simulink model "EV_thermal_charger_2015a_jmaab_Can01"  (R2015a)
settings: Solver=ode3  StartTime=0.0  StopTime=1800  FixedStep=sampling_time  RelTol=1e-3
PreLoadFcn:
  | %run('init_setting.m')
PostLoadFcn:
  | %set_param(gcs, 'SimulationCommand', 'update');
  | %load('save_param/save_P_Charger', 'P_Charger');
  | %load('save_param/save_T_User_set_temp_degC','T_User_set_temp_degC');
  | %load('save_param/save_ENV_PNT_PTTH_Temp_add_degC','ENV_PNT_PTTH_Temp_add_degC');
  | %load('save_param/save_ENV_PNT_CABIN_Temp_add_degC','ENV_PNT_CABIN_Temp_add_degC');
  | %load('save_param/save_ENV_PNT_PHI_Sunlight_W','ENV_PNT_PHI_Sunlight_W');
  | %load('save_param/save_ENV_PNT_Outside_Temp_ini_degC','ENV_PNT_Outside_Temp_ini_degC');
undefined symbols (not defined in the file or in its folder): BK_PNT_Pow_UL, BK_PNT_ReGene_vel_limit_DN_kmph, BK_PNT_ReGene_vel_limit_UP_kmph, BK_PNT_Tau_brake, Brk_LL, Brk_PGain, Brk_UL, BT_PNT_Hi_C_pol_hi_batt, BT_PNT_Hi_Capa_hi_batt_F, BT_PNT_Hi_ocv_SOC_hi_batt_OCV_V_table, BT_PNT_Hi_ocv_SOC_hi_batt_OCV_V_table_x_SOC, BT_PNT_Hi_R_hi_batt_cell, BT_PNT_Hi_R_pol_hi_batt, BT_PNT_Hi_SOC_MAX_hi_batt, BT_PNT_Hi_SOC_MIN_hi_batt, BT_PNT_Hi_SOC_START_hi_batt, BT_PNT_Lo_Capa_lo_batt_F, BT_PNT_Lo_ocv_SOC_lo_batt_OCV_V_table, BT_PNT_Lo_ocv_SOC_lo_batt_OCV_V_table_x_SOC, BT_PNT_Lo_R_lo_batt_ohm, BT_PNT_Lo_SOC_MAX_lo_batt, BT_PNT_Lo_SOC_MIN_lo_batt, BT_PNT_Lo_SOC_START_lo_batt, BTTH_CNT_P_BT_Heater_W, BTTH_CNT_P_BT_Heater_W_x_BTCells_degC, BTTH_CNT_Voltage_BTFan_V, BTTH_CNT_Voltage_BTFan_V_x_BTCells_degC, BTTH_PNT_BT_Heat_Resi_KpW, BTTH_PNT_BT_Heat_Resi_KpW_x_Wind_m3ps, BTTH_PNT_BT_Heater2BTCells_Heat_Resi_KpW, BTTH_PNT_BT_Heater_Heat_Capa_JpK, BTTH_PNT_BTBlock2BTAir_Heat_Resi_KpW, BTTH_PNT_BTBlock_Heat_Capa_JpK, BTTH_PNT_BTCells2BTBlock_Heat_Resi_KpW, BTTH_PNT_BTCells_Heat_Capa_JpK, BTTH_PNT_v_BTFan_Wind_vel_mps, BTTH_PNT_v_BTFan_Wind_vel_mps_x_V_BTFan, CATH_CNT_P_Aircon_W_LL, CATH_CNT_P_Aircon_W_UL, CATH_CNT_P_Gain_Aircon, CATH_CNT_P_Gain_PTC_Heater, CATH_CNT_P_Gain_SeatHT, CATH_CNT_P_PTC_Heater, CATH_CNT_P_PTC_Heater_W_LL, CATH_CNT_P_PTC_Heater_W_UL, CATH_CNT_P_PTC_Heater_x_T_Outside_temp_degC, CATH_CNT_P_SeatHT_W_LL, CATH_CNT_P_SeatHT_W_UL, CATH_CNT_PGain_Temp_blowout, CATH_CNT_T_Aircon_Indoor_degC, CATH_CNT_T_Aircon_Indoor_degC_x_T_blowout_degC, CATH_CNT_T_PTC_Heater_degC_UL, CATH_CNT_T_SeatHT_Temp_degC, CATH_CNT_T_SeatHT_Temp_degC_x_T_blowout_degC, CATH_CNT_V_HVAC_Fan, CATH_CNT_V_HVAC_Fan_x_T_blowout_degC, CATH_CNT_V_RDFan_V, CATH_CNT_V_RDFan_x_P_Aircon_W, CATH_PNT_Air_Convection_Heat_Resi_KpW, CATH_PNT_Air_Convection_Heat_Resi_x_mps ... (+141)
undefined symbols (not defined in the file): ACC_D_Gain, ACC_I_Gain, ACC_P_Gain
libraries: METI_Lib_vehicle_model x52, simulink x35
(part 5 of 6)

== system EV_thermal_charger_2015a_jmaab_Can01/Vehicle/CNT/VCU_CNT/VCU_CNT/PDfSOC ==
  note: 放電電力マップ
  note: 充電電力マップ
  SOC_BT_Hi_PNT_per : Inport
  PSoFin_map : Lookup_n-D  NumberOfTableDimensions=1  BreakpointsForDimension1=VCU_CNT_PSoFin_soc  BeginIndexSearchUsingPreviousIndexResult=on  Table=VCU_CNT_PSoFin_battpw  ExtrapMethod=Clip  UseLastTableValue=on  InternalRulePriority=Speed  RndMeth=Simplest  InputSameDT=on
  PSoFout_map : Lookup_n-D  NumberOfTableDimensions=1  BreakpointsForDimension1=VCU_CNT_PSoFout_soc  BeginIndexSearchUsingPreviousIndexResult=on  Table=VCU_CNT_PSoFout_battpw  ExtrapMethod=Clip  UseLastTableValue=on  InternalRulePriority=Speed  RndMeth=Simplest  InputSameDT=on
  PSoFin : Outport
  PSoFout : Outport  Port=2
  wires:
  PSoFout_map/1 -> PSoFout/1
  PSoFin_map/1 -> PSoFin/1
  SOC_BT_Hi_PNT_per/1 -> PSoFout_map/1, PSoFin_map/1

== system EV_thermal_charger_2015a_jmaab_Can01/Vehicle/CNT/VCU_CNT/VCU_CNT/ReGenerativeBrake_Calc ==
  note: 回生ブレーキ
      | 推進力[N]
  note: 回生ブレーキ
      | モータートルク[N]
  v_VL_PNT_kmph : Inport
  open_break_Driver_per : Inport  Port=2
  Constant : Constant  Value=0
  Constant2 : Constant  Value=1/TM_PNT_ratio_MG2_gear
  Constant4 : Constant  Value=tire_r
  Constant5 : Constant  Value=BK_PNT_Pow_UL
  Constant9 : Constant  Value=1/DF_PNT_DF_gear
  Gain : Gain  Gain=-1
  Product1 : Product  Inputs=6
  Product2 : Product
  ReBrake_Limit_Lowspeed : Subsystem
  Saturation Dynamic : simulink/Discontinuities/Saturation Dynamic  OutMin=[]  OutMax=[]  OutDataTypeStr=Inherit: Same as second input  OutDataType=fixdt(1, 16)  OutScaling=2^-10  DoSatur=off
  eta_DF1 : Constant  Value=TM_PNT_eta_MG2_gear
  eta_DF2 : Constant  Value=DF_PNT_eta_DF
  per2F2 : Gain  Gain=1/100
  trq_R_brake_tgt : Outport
  wires:
  Saturation Dynamic/1 -> Product1/1
  Constant/1 -> Saturation Dynamic/1
  Gain/1 -> Saturation Dynamic/2
  per2F2/1 -> Product2/1
  Constant5/1 -> Product2/2
  Product2/1 -> Gain/1
  open_break_Driver_per/1 -> per2F2/1
  Constant4/1 -> Product1/2
  Constant9/1 -> Product1/3
  eta_DF2/1 -> Product1/4
  Product1/1 -> trq_R_brake_tgt/1
  Constant2/1 -> Product1/5
  eta_DF1/1 -> Product1/6
  v_VL_PNT_kmph/1 -> ReBrake_Limit_Lowspeed/1(v_VL_PNT_kmph)
  ReBrake_Limit_Lowspeed/1(F_Brake_limit_lowspeed) -> Saturation Dynamic/3

== system EV_thermal_charger_2015a_jmaab_Can01/Vehicle/CNT/VCU_CNT/VCU_CNT/trq_MG2_GuardCalc ==
  note: 回生側のトルク制限
  note: 加速側のトルク制限
  w_MG_PNT_radps : Inport
  PSoFin : Inport  Port=2
  PSoFout : Inport  Port=3
  P_HVAC_PNT_W : Inport  Port=4
  P_DCDC_PNT_W : Inport  Port=5
  Abs : Abs
  Divide_0wari : METI_Lib_vehicle_model/Divide_0wari
  Divide_0wari1 : METI_Lib_vehicle_model/Divide_0wari
  MinMax : MinMax  Function=max  Inputs=2
  MinMax1 : MinMax  Inputs=2
  MinMax2 : MinMax  Inputs=2
  MinMax3 : MinMax  Function=max  Inputs=2
  Subtract1 : Sum  Inputs=+--
  Subtract2 : Sum  Inputs=+--
  力行側出力上限 : Constant  Value=MG_CNT_Pmax_MG_Gene_W
  力行側定トルク回転数上限 : Constant  Value=MG_CNT_MG_Const_trq_Gene_radps
  回生側出力上限 : Constant  Value=MG_CNT_Pmin_MG_ReGene_W
  回生側定トルク回転数上限 : Constant  Value=MG_CNT_MG_Const_trq_ReGene_radps
  trq_MG2_UpperGuard : Outport
  trq_MG2_LowerGuard : Outport  Port=2
  wires:
  MinMax2/1 -> Divide_0wari1/1  "使用可能電力"
  w_MG_PNT_radps/1 -> Abs/1
  Divide_0wari1/1 -> trq_MG2_UpperGuard/1  "トルク上限"
  MinMax/1 -> Divide_0wari1/2, Divide_0wari/2
  Abs/1 -> MinMax/1
  MinMax1/1 -> MinMax/2
  PSoFout/1 -> Subtract1/1  "バッテリ放電電力上限値"
  P_HVAC_PNT_W/1 -> Subtract2/2, Subtract1/2
  MinMax3/1 -> Divide_0wari/1
  Divide_0wari/1 -> trq_MG2_LowerGuard/1
  PSoFin/1 -> Subtract2/1
  力行側定トルク回転数上限/1 -> MinMax1/1
  回生側定トルク回転数上限/1 -> MinMax1/2
  Subtract1/1 -> MinMax2/1  "使用可能電力"
  Subtract2/1 -> MinMax3/2
  力行側出力上限/1 -> MinMax2/2
  回生側出力上限/1 -> MinMax3/1
  P_DCDC_PNT_W/1 -> Subtract2/3, Subtract1/3

== system EV_thermal_charger_2015a_jmaab_Can01/Vehicle/CNT/VCU_CNT/VCU_CNT/trq_MG2_tgtCalc2 ==
  note: ～回生協調ブレーキ時～
      | アクセルオフによる回生ブレーキトルクと
      | ブレーキ操作による回生ブレーキトルクを合算し
      | モーター要求トルクとする
  note: ～回生協調ブレーキ時～
      | モーター要求トルクから
      | アクセルオフによる回生ブレーキトルクを減算し
      | 実際に出力できているブレーキ操作による回生ブレーキトルクを算出
      | それを車両駆動力としてブレーキECUへ送信する
  User_Power_req : Inport
  w_MG_PNT_radps : Inport  Port=2
  trq_motor_UserAcc_tgt : Inport  Port=3
  trq_MG2_UpperGuard : Inport  Port=4
  trq_MG2_LowerGuard : Inport  Port=5
  trq_R_brake_tgt : Inport  Port=6
  Add : Sum
  Add1 : Sum  Inputs=+-
  Constant1 : Constant  Value=TM_PNT_ratio_MG2_gear
  Constant2 : Constant  Value=DF_PNT_DF_gear
  Constant4 : Constant  Value=1/tire_r
  Product1 : Product  Inputs=6
  Saturation Dynamic2 : simulink/Discontinuities/Saturation Dynamic  OutMin=[]  OutMax=[]  OutDataTypeStr=Inherit: Same as second input  OutDataType=fixdt(1, 16)  OutScaling=2^-10  DoSatur=off
  Saturation Dynamic4 : simulink/Discontinuities/Saturation Dynamic  OutMin=[]  OutMax=[]  OutDataTypeStr=Inherit: Same as second input  OutDataType=fixdt(1, 16)  OutScaling=2^-10  DoSatur=off
  Switch4 : Switch  Criteria=u2 > Threshold
  eta_DF1 : Constant  Value=1/DF_PNT_eta_DF
  eta_DF2 : Constant  Value=1/TM_PNT_eta_MG2_gear
  回転数上限超過時トルク制限処理 : Subsystem
  tgt_Trq_VCU_CNT_MG_Nm : Outport
  F_VCU_CNT_re_break_N : Outport  Port=2
  wires:
  Saturation Dynamic4/1 -> Add1/1, tgt_Trq_VCU_CNT_MG_Nm/1
  trq_MG2_LowerGuard/1 -> Saturation Dynamic2/3, Saturation Dynamic4/3
  回転数上限超過時トルク制限処理/1(flag_overrev) -> Switch4/2
  Add/1 -> Saturation Dynamic4/2
  trq_motor_UserAcc_tgt/1 -> 回転数上限超過時トルク制限処理/1(trq_MG2_tgt), Switch4/1
  trq_MG2_UpperGuard/1 -> Saturation Dynamic2/1, Saturation Dynamic4/1
  w_MG_PNT_radps/1 -> 回転数上限超過時トルク制限処理/2(w_ROT_motor)
  User_Power_req/1 -> 回転数上限超過時トルク制限処理/3(User_Power_req)
  回転数上限超過時トルク制限処理/2(trq_MG2_guarded) -> Switch4/3
  Add1/1 -> Product1/1
  Constant4/1 -> Product1/2
  Constant2/1 -> Product1/3
  eta_DF1/1 -> Product1/4
  Product1/1 -> F_VCU_CNT_re_break_N/1
  Switch4/1 -> Add/2, Saturation Dynamic2/2
  trq_R_brake_tgt/1 -> Add/1
  Saturation Dynamic2/1 -> Add1/2
  Constant1/1 -> Product1/5
  eta_DF2/1 -> Product1/6

== system EV_thermal_charger_2015a_jmaab_Can01/Vehicle/CNT/VCU_CNT/VCU_CNT/ユーザ要求駆力算出 ==
  note: 低速時に目標出力が0にならないよう
      | 5km/h以下では車速を5km/hとして
      | 目標出力を計算するための
      | 速度切替処理
  note: モーター軸の要求トルク
  open_accel_Driver_per : Inport
  open_break_Driver_per : Inport  Port=2
  v_VL_PNT_kmph : Inport  Port=3
  Compare To Constant : simulink/Logic and Bit Operations/Compare To Constant  relop=<  const=VCU_CNT_trq_req_v_vehicle_th  OutDataTypeStr=boolean
  Compare To Constant1 : simulink/Logic and Bit Operations/Compare To Constant  relop=>  const=VCU_CNT_trq_req_brak_th  OutDataTypeStr=boolean
  Constant : Constant  Value=5
  Constant1 : Constant  Value=DF_PNT_DF_gear
  Constant2 : Constant  Value=TM_PNT_ratio_MG2_gear
  Constant3 : Constant  Value=VCU_CNT_trq_req_Gain_ON
  Constant4 : Constant  Value=1/tire_r
  Constant5 : Constant  Value=VCU_CNT_trq_req_Gain_OFF
  Gain1 : Gain  Commented=through  Gain=mps2kmph
  Logical Operator : Logic  AllPortsSameDT=off  OutDataTypeStr=boolean
  Product : Product
  Product1 : Product  Inputs=6
  Product3 : Product
  Relational Operator : RelationalOperator  Operator=>  OutDataTypeStr=boolean
  Switch : Switch  Criteria=u2 > Threshold  Threshold=0.5
  Switch1 : Switch  Criteria=u2 > Threshold  Threshold=0.5
  Transfer Fcn : TransferFcn  Denominator=[VCU_CNT_trq_req_delaytime 1]
  eta_DF1 : Constant  Value=DF_PNT_eta_DF
  eta_DF2 : Constant  Value=TM_PNT_eta_MG2_gear
  kmph2mps : Gain  Gain=kmph2mps
  kmph2mps1 : Gain  Commented=through  Gain=kmph2mps
  mps2kmph : Gain  Commented=through  Gain=mps2kmph
  要求駆動トルク推定 : Lookup_n-D  BreakpointsForDimension1=VCU_CNT_trq_require_v_kmph  BreakpointsForDimension2=VCU_CNT_trq_require_accper  BeginIndexSearchUsingPreviousIndexResult=on  Table=VCU_CNT_trq_require_Nm  ExtrapMethod=Clip  InternalRulePriority=Speed  RndMeth=Simplest  InputSameDT=on
  P_vehicle_tgt : Outport
  trq_motor_UserAcc_tgt : Outport  Port=2
  wires:
  Switch/1 -> kmph2mps/1
  Product3/1 -> P_vehicle_tgt/1
  Constant/1 -> kmph2mps1/1, Relational Operator/2
  mps2kmph/1 -> Relational Operator/1
  Relational Operator/1 -> Switch/2
  kmph2mps1/1 -> Switch/3
  Constant4/1 -> Product1/1
  Constant1/1 -> Product1/2
  eta_DF1/1 -> Product1/3
  Product1/1 -> Product3/2
  要求駆動トルク推定/1 -> Product1/6, Product/1
  Constant5/1 -> Switch1/1
  v_VL_PNT_kmph/1 -> mps2kmph/1, Gain1/1, Switch/1
  open_break_Driver_per/1 -> Compare To Constant1/1
  Compare To Constant/1 -> Logical Operator/1
  Compare To Constant1/1 -> Logical Operator/2
  Logical Operator/1 -> Switch1/2
  Constant3/1 -> Switch1/3
  Switch1/1 -> Transfer Fcn/1
  Transfer Fcn/1 -> Product/2
  Product/1 -> trq_motor_UserAcc_tgt/1
  Gain1/1 -> 要求駆動トルク推定/1, Compare To Constant/1
  open_accel_Driver_per/1 -> 要求駆動トルク推定/2
  Constant2/1 -> Product1/4
  eta_DF2/1 -> Product1/5
  kmph2mps/1 -> Product3/1

== system EV_thermal_charger_2015a_jmaab_Can01/Vehicle/DTTH/DTTH_PNT/DFTH_PNT/DFBlock2Air_Heat_Resistance ==
  "T_DFBlock_Resi3_K " : Inport
  T_DF_Air_Resi1_K : Inport  Port=2
  Add : Sum  Inputs=+-
  Constant : Constant  Value=PTTH_PNT_DFBlock2DFAir_Heat_Resi_KpW
  Divide : Product  Inputs=*/
  Gain : Gain  Gain=-1
  Gain1 : Gain
  "PHI_DF_Air_Resi1_W " : Outport
  "PHI_DFBlock_Resi3_W " : Outport  Port=2
  wires:
  Constant/1 -> Divide/2
  Add/1 -> Divide/1
  Divide/1 -> Gain/1, Gain1/1
  "T_DFBlock_Resi3_K "/1 -> Add/1
  Gain1/1 -> "PHI_DF_Air_Resi1_W "/1
  T_DF_Air_Resi1_K/1 -> Add/2
  Gain/1 -> "PHI_DFBlock_Resi3_W "/1

== system EV_thermal_charger_2015a_jmaab_Can01/Vehicle/DTTH/DTTH_PNT/DFTH_PNT/DFBlock_Heat_Capacity ==
  Temp_ini : Inport
  "PHI_DFBlock1_W " : Inport  Port=2
  "PHI_DFBlock2_W " : Inport  Port=3
  PHI_DFBlock3_W : Inport  Port=4
  Add : Sum  Inputs=+++
  Add1 : Sum
  Constant : Constant  Value=PTTH_PNT_DFBlock_Heat_Capa_JpK
  Divide : Product  Inputs=/*
  Integrator : Integrator
  degC->K : Subsystem
  "T_DFBlock1_K " : Outport
  T_DFBlock2_K : Outport  Port=2
  "T_DFBlock3_K " : Outport  Port=3
  wires:
  "PHI_DFBlock1_W "/1 -> Add/1
  Constant/1 -> Divide/1
  Add/1 -> Divide/2
  Divide/1 -> Integrator/1
  Temp_ini/1 -> degC->K/1(degC)
  Integrator/1 -> Add1/2
  Add1/1 -> "T_DFBlock3_K "/1, "T_DFBlock1_K "/1, T_DFBlock2_K/1
  "PHI_DFBlock2_W "/1 -> Add/2
  PHI_DFBlock3_W/1 -> Add/3
  degC->K/1(K) -> Add1/1

== system EV_thermal_charger_2015a_jmaab_Can01/Vehicle/DTTH/DTTH_PNT/DFTH_PNT/DFOil2DFBlock_Heat_Resistance ==
  T_DFBlock_Resi1_K : Inport
  "T_DFOil_Resi2_K " : Inport  Port=2
  Add : Sum  Inputs=+-
  Constant : Constant  Value=PTTH_PNT_DFOil2DFBlock_Heat_Resi_KpW
  Divide : Product  Inputs=*/
  Gain : Gain  Gain=-1
  Gain1 : Gain
  PHI_DFBlock_Resi1_W : Outport
  PHI_DFOil_Resi2_W : Outport  Port=2
  wires:
  Constant/1 -> Divide/2
  Add/1 -> Divide/1
  Divide/1 -> Gain1/1, Gain/1
  Gain/1 -> PHI_DFOil_Resi2_W/1
  "T_DFOil_Resi2_K "/1 -> Add/1
  T_DFBlock_Resi1_K/1 -> Add/2
  Gain1/1 -> PHI_DFBlock_Resi1_W/1

== system EV_thermal_charger_2015a_jmaab_Can01/Vehicle/DTTH/DTTH_PNT/DFTH_PNT/DFOil_Heat_Capacity ==
  Temp_ini : Inport
  PHI_DFOil1_W : Inport  Port=2
  "PHI_DFOil2_W " : Inport  Port=3
  Add : Sum
  Add1 : Sum
  Constant : Constant  Value=PTTH_PNT_DFOil_Heat_Capa_JpK
  Divide : Product  Inputs=/*
  Integrator : Integrator
  degC->K : Subsystem
  "T_DFOil1_K " : Outport
  T_DFOil2_K : Outport  Port=2
  wires:
  "PHI_DFOil2_W "/1 -> Add/2
  PHI_DFOil1_W/1 -> Add/1
  Constant/1 -> Divide/1
  Add/1 -> Divide/2
  Divide/1 -> Integrator/1
  Temp_ini/1 -> degC->K/1(degC)
  Integrator/1 -> Add1/2
  Add1/1 -> T_DFOil2_K/1, "T_DFOil1_K "/1
  degC->K/1(K) -> Add1/1

== system EV_thermal_charger_2015a_jmaab_Can01/Vehicle/DTTH/DTTH_PNT/DFTH_PNT/K->degC1 ==
  K : Inport
  Constant2 : Constant  Value=K2degC
  Sum : Sum  Inputs=++|
  degC : Outport
  wires:
  K/1 -> Sum/2
  Constant2/1 -> Sum/1
  Sum/1 -> degC/1

== system EV_thermal_charger_2015a_jmaab_Can01/Vehicle/DTTH/DTTH_PNT/DFTH_PNT/TMBlock2DFBlock_Heat_Resistance ==
  "T_DFBlock_Resi2_K " : Inport
  "T_TMBlock_Resi4_K " : Inport  Port=2
  Add : Sum  Inputs=+-
  Constant : Constant  Value=PTTH_PNT_TMBlock2DFBlock_Heat_Resi_KpW
  Divide : Product  Inputs=*/
  Gain : Gain  Gain=-1
  Gain1 : Gain
  "PHI_DFBlock_Resi2_W " : Outport
  "PHI_TMBlock_Resi4_W " : Outport  Port=2
  wires:
  Constant/1 -> Divide/2
  Add/1 -> Divide/1
  Divide/1 -> Gain/1, Gain1/1
  Gain/1 -> "PHI_TMBlock_Resi4_W "/1
  "T_TMBlock_Resi4_K "/1 -> Add/1
  "T_DFBlock_Resi2_K "/1 -> Add/2
  Gain1/1 -> "PHI_DFBlock_Resi2_W "/1

== system EV_thermal_charger_2015a_jmaab_Can01/Vehicle/DTTH/DTTH_PNT/TMTH_PNT/K->degC1 ==
  K : Inport
  Constant2 : Constant  Value=K2degC
  Sum : Sum  Inputs=++|
  degC : Outport
  wires:
  K/1 -> Sum/2
  Constant2/1 -> Sum/1
  Sum/1 -> degC/1

== system EV_thermal_charger_2015a_jmaab_Can01/Vehicle/DTTH/DTTH_PNT/TMTH_PNT/TF2TMBlock_Heat_Resistance ==
  "T_TMBlock_Resi1_K " : Inport
  "T_TF_Resi2_K " : Inport  Port=2
  Add : Sum  Inputs=+-
  Constant : Constant  Value=PTTH_PNT_TF2TMBlock_Heat_Resi_KpW
  Divide : Product  Inputs=*/
  Gain : Gain  Gain=-1
  Gain1 : Gain
  PHI_TMBlock_Resi1_W : Outport
  PHI_TF_Resi2_W : Outport  Port=2
  wires:
  Constant/1 -> Divide/2
  Add/1 -> Divide/1
  Divide/1 -> Gain/1, Gain1/1
  Gain/1 -> PHI_TF_Resi2_W/1
  "T_TF_Resi2_K "/1 -> Add/1
  "T_TMBlock_Resi1_K "/1 -> Add/2
  Gain1/1 -> PHI_TMBlock_Resi1_W/1

== system EV_thermal_charger_2015a_jmaab_Can01/Vehicle/DTTH/DTTH_PNT/TMTH_PNT/TF_Heat_Capacity ==
  Temp_ini : Inport
  PHI_TF1_W : Inport  Port=2
  PHI_TF2_W : Inport  Port=3
  Add : Sum
  Add1 : Sum
  Constant : Constant  Value=PTTH_PNT_TF_Heat_Capa_JpK
  Divide : Product  Inputs=/*
  Integrator : Integrator
  degC->K : Subsystem
  T_TF1_K : Outport
  T_TF2_K : Outport  Port=2
  wires:
  PHI_TF1_W/1 -> Add/1
  Constant/1 -> Divide/1
  Add/1 -> Divide/2
  Divide/1 -> Integrator/1
  Temp_ini/1 -> degC->K/1(degC)
  Integrator/1 -> Add1/2
  Add1/1 -> T_TF2_K/1, T_TF1_K/1
  PHI_TF2_W/1 -> Add/2
  degC->K/1(K) -> Add1/1

== system EV_thermal_charger_2015a_jmaab_Can01/Vehicle/DTTH/DTTH_PNT/TMTH_PNT/TMBlock2Air_Heat_Resistance ==
  T_TM_Air_Resi1_K : Inport
  "T_TMBlock_Resi3_K " : Inport  Port=2
  Add : Sum  Inputs=+-
  Constant : Constant  Value=PTTH_PNT_TMBlock2TMAir_Heat_Resi_KpW
  Divide : Product  Inputs=*/
  Gain : Gain  Gain=-1
  Gain1 : Gain
  "PHI_TM_Air_Resi1_W " : Outport
  PHI_TMBlock_Resi3_W : Outport  Port=2
  wires:
  Constant/1 -> Divide/2
  Add/1 -> Divide/1
  Divide/1 -> Gain/1, Gain1/1
  Gain/1 -> PHI_TMBlock_Resi3_W/1
  "T_TMBlock_Resi3_K "/1 -> Add/1
  Gain1/1 -> "PHI_TM_Air_Resi1_W "/1
  T_TM_Air_Resi1_K/1 -> Add/2

== system EV_thermal_charger_2015a_jmaab_Can01/Vehicle/DTTH/DTTH_PNT/TMTH_PNT/TMBlock_Heat_Capacity ==
  Temp_ini : Inport
  PHI_TMBlock1_W : Inport  Port=2
  PHI_TMBlock2_W : Inport  Port=3
  PHI_TMBlock3_W : Inport  Port=4
  PHI_TMBlock4_W : Inport  Port=5
  Add : Sum  Inputs=++++
  Add1 : Sum
  Constant : Constant  Value=PTTH_PNT_TMBlock_Heat_Capa_JpK
  Divide : Product  Inputs=/*
  Integrator : Integrator
  degC->K : Subsystem
  T_TMBlock1_K : Outport
  T_TMBlock2_K : Outport  Port=2
  T_TMBlock3_K : Outport  Port=3
  T_TMBlock4_K : Outport  Port=4
  wires:
  PHI_TMBlock1_W/1 -> Add/1
  Constant/1 -> Divide/1
  Add/1 -> Divide/2
  Divide/1 -> Integrator/1
  Temp_ini/1 -> degC->K/1(degC)
  Integrator/1 -> Add1/2
  Add1/1 -> T_TMBlock4_K/1, T_TMBlock3_K/1, T_TMBlock1_K/1, T_TMBlock2_K/1
  PHI_TMBlock3_W/1 -> Add/3
  PHI_TMBlock2_W/1 -> Add/2
  degC->K/1(K) -> Add1/1
  PHI_TMBlock4_W/1 -> Add/4

== system EV_thermal_charger_2015a_jmaab_Can01/Vehicle/ELTH/ELTH_PNT/INVTH_PNT/INVBlock2Air_Heat_Resistance ==
  T_INV2Air_Resi1_K : Inport
  T_INVBlock_Resi3_K : Inport  Port=2
  Add : Sum  Inputs=+-
  Constant : Constant  Value=ELTH_PNT_INVBlock2DFAir_Heat_Resi_KpW
  Divide : Product  Inputs=*/
  Gain : Gain  Gain=-1
  Gain1 : Gain
  PHI_INV2Air_Resi1_W : Outport
  PHI_INVBlock_Resi3_W : Outport  Port=2
  wires:
  Constant/1 -> Divide/2
  Add/1 -> Divide/1
  Divide/1 -> Gain1/1, Gain/1
  Gain/1 -> PHI_INVBlock_Resi3_W/1
  T_INVBlock_Resi3_K/1 -> Add/1
  T_INV2Air_Resi1_K/1 -> Add/2
  Gain1/1 -> PHI_INV2Air_Resi1_W/1

== system EV_thermal_charger_2015a_jmaab_Can01/Vehicle/ELTH/ELTH_PNT/INVTH_PNT/INVBlock_Heat_Capacity ==
  PHI_INVBlock2_W : Inport
  Temp_ini : Inport  Port=2
  PHI_INVBlock1_W : Inport  Port=3
  PHI_INVBlock3_W : Inport  Port=4
  Add : Sum  Inputs=+++
  Add1 : Sum
  Constant : Constant  Value=ELTH_PNT_INVBlock_Heat_Capa_JpK
  Divide : Product  Inputs=/*
  Integrator : Integrator
  degC->K : Subsystem
  T_INVBlock2_K : Outport
  T_INVBlock3_K : Outport  Port=2
  T_INVBlock1_K : Outport  Port=3
  wires:
  PHI_INVBlock1_W/1 -> Add/1
  Constant/1 -> Divide/1
  Add/1 -> Divide/2
  Divide/1 -> Integrator/1
  Temp_ini/1 -> degC->K/1(degC)
  Integrator/1 -> Add1/2
  Add1/1 -> T_INVBlock3_K/1, T_INVBlock2_K/1, T_INVBlock1_K/1
  PHI_INVBlock2_W/1 -> Add/2
  PHI_INVBlock3_W/1 -> Add/3
  degC->K/1(K) -> Add1/1

== system EV_thermal_charger_2015a_jmaab_Can01/Vehicle/ELTH/ELTH_PNT/INVTH_PNT/INVHeatsink2INVBlock_Heat_Resistance ==
  T_INVHeatsink_Resi2_K : Inport
  T_INVBlock_Resi1_K : Inport  Port=2
  Add : Sum  Inputs=+-
  Constant : Constant  Value=ELTH_PNT_INVHeatsink2INVBlock_Heat_Resi_KpW
  Divide : Product  Inputs=*/
  Gain : Gain  Gain=-1
  Gain1 : Gain
  PHI_INVBlock_Resi1_W : Outport
  PHI_INVHeatsink_Resi2_W : Outport  Port=2
  wires:
  Constant/1 -> Divide/2
  Add/1 -> Divide/1
  Divide/1 -> Gain1/1, Gain/1
  Gain/1 -> PHI_INVHeatsink_Resi2_W/1
  T_INVHeatsink_Resi2_K/1 -> Add/1
  T_INVBlock_Resi1_K/1 -> Add/2
  Gain1/1 -> PHI_INVBlock_Resi1_W/1

== system EV_thermal_charger_2015a_jmaab_Can01/Vehicle/ELTH/ELTH_PNT/INVTH_PNT/INVTH_Heatsink_Heat_Capacity ==
  Temp_ini : Inport
  PHI_INVTH_Heatsink1_W : Inport  Port=2
  PHI_INVTH_Heatsink3_W : Inport  Port=3
  PHI_INVTH_Heatsink2_W : Inport  Port=4
  Add : Sum  Inputs=+++
  Add1 : Sum
  Constant : Constant  Value=ELTH_PNT_INVHeatsink_Heat_Capa_JpK
  Divide : Product  Inputs=/*
  Integrator : Integrator
  degC->K : Subsystem
  T_INVTH_Heatsink1_K : Outport
  T_INVTH_Heatsink2_K : Outport  Port=2
  T_INVTH_Heatsink3_K : Outport  Port=3
  wires:
  PHI_INVTH_Heatsink2_W/1 -> Add/3
  PHI_INVTH_Heatsink1_W/1 -> Add/1
  Constant/1 -> Divide/1
  Add/1 -> Divide/2
  Divide/1 -> Integrator/1
  Temp_ini/1 -> degC->K/1(degC)
  Integrator/1 -> Add1/2
  Add1/1 -> T_INVTH_Heatsink3_K/1, T_INVTH_Heatsink2_K/1, T_INVTH_Heatsink1_K/1
  degC->K/1(K) -> Add1/1
  PHI_INVTH_Heatsink3_W/1 -> Add/2

== system EV_thermal_charger_2015a_jmaab_Can01/Vehicle/ELTH/ELTH_PNT/INVTH_PNT/K->degC1 ==
  K : Inport
  Constant2 : Constant  Value=K2degC
  Sum : Sum  Inputs=++|
  degC : Outport
  wires:
  K/1 -> Sum/2
  Constant2/1 -> Sum/1
  Sum/1 -> degC/1

== system EV_thermal_charger_2015a_jmaab_Can01/Vehicle/ELTH/ELTH_PNT/INVTH_PNT/K->degC2 ==
  K : Inport
  Constant2 : Constant  Value=K2degC
  Sum : Sum  Inputs=++|
  degC : Outport
  wires:
  K/1 -> Sum/2
  Constant2/1 -> Sum/1
  Sum/1 -> degC/1

== system EV_thermal_charger_2015a_jmaab_Can01/Vehicle/ELTH/ELTH_PNT/INVTH_PNT/MG2INVBlock_Heat_Resistance ==
  T_INVBlock_Resi2_K : Inport
  T_MGBlock_Resi4_K : Inport  Port=2
  Add : Sum  Inputs=+-
  Constant : Constant  Value=ELTH_PNT_MG2INVBlock_Heat_Resi_KpW
  Divide : Product  Inputs=*/
  Gain : Gain  Gain=-1
  Gain1 : Gain
  PHI_INVBlock_Resi2_W : Outport
  PHI_MGBlock_Resi4_W : Outport  Port=2
  wires:
  Constant/1 -> Divide/2
  Add/1 -> Divide/1
  Divide/1 -> Gain1/1, Gain/1
  Gain/1 -> PHI_MGBlock_Resi4_W/1
  T_MGBlock_Resi4_K/1 -> Add/1
  T_INVBlock_Resi2_K/1 -> Add/2
  Gain1/1 -> PHI_INVBlock_Resi2_W/1

== system EV_thermal_charger_2015a_jmaab_Can01/Vehicle/ELTH/ELTH_PNT/MGTH_PNT/Coil_Heat_Capacity ==
  Temp_ini : Inport
  PHI_MGCoil1_W : Inport  Port=2
  PHI_MGCoil2_W : Inport  Port=3
  Add : Sum
  Add1 : Sum
  Constant : Constant  Value=ELTH_PNT_MGCoil_Heat_Capa_JpK
  Divide : Product  Inputs=/*
  Integrator : Integrator
  degC->K : Subsystem
  T_MGCoil1_K : Outport
  T_MGCoil2_K : Outport  Port=2
  wires:
  PHI_MGCoil2_W/1 -> Add/2
  PHI_MGCoil1_W/1 -> Add/1
  Constant/1 -> Divide/1
  Add/1 -> Divide/2
  Divide/1 -> Integrator/1
  Temp_ini/1 -> degC->K/1(degC)
  Integrator/1 -> Add1/2
  Add1/1 -> T_MGCoil1_K/1, T_MGCoil2_K/1
  degC->K/1(K) -> Add1/1

== system EV_thermal_charger_2015a_jmaab_Can01/Vehicle/ELTH/ELTH_PNT/MGTH_PNT/K->degC1 ==
  K : Inport
  Constant2 : Constant  Value=K2degC
  Sum : Sum  Inputs=++|
  degC : Outport
  wires:
  K/1 -> Sum/2
  Constant2/1 -> Sum/1
  Sum/1 -> degC/1

== system EV_thermal_charger_2015a_jmaab_Can01/Vehicle/ELTH/ELTH_PNT/MGTH_PNT/K->degC2 ==
  K : Inport
  Constant2 : Constant  Value=K2degC
  Sum : Sum  Inputs=++|
  degC : Outport
  wires:
  K/1 -> Sum/2
  Constant2/1 -> Sum/1
  Sum/1 -> degC/1

== system EV_thermal_charger_2015a_jmaab_Can01/Vehicle/ELTH/ELTH_PNT/MGTH_PNT/MGCoil2MGHousing_Heat_Resistance ==
  T_MGCoil_Resi4_K : Inport
  T_MGHousing_Resi1_K : Inport  Port=2
  Add : Sum  Inputs=+-
  Constant : Constant  Value=ELTH_PNT_MGCoil2MGHousing_Heat_Resi_KpW
  Divide : Product  Inputs=*/
  Gain : Gain  Gain=-1
  Gain1 : Gain
  PHI_MGHousing_Resi1_W : Outport
  PHI_MGCoil_Resi4_W : Outport  Port=2
  wires:
  Constant/1 -> Divide/2
  Add/1 -> Divide/1
  Divide/1 -> Gain/1, Gain1/1
  Gain/1 -> PHI_MGCoil_Resi4_W/1
  T_MGCoil_Resi4_K/1 -> Add/1
  T_MGHousing_Resi1_K/1 -> Add/2
  Gain1/1 -> PHI_MGHousing_Resi1_W/1

== system EV_thermal_charger_2015a_jmaab_Can01/Vehicle/ELTH/ELTH_PNT/MGTH_PNT/MGHousing2Air_Heat_Resistance ==
  T_MG2Air_Resi1_K : Inport
  T_MGHousing_Resi5_K : Inport  Port=2
  Add : Sum  Inputs=+-
  Constant : Constant  Value=ELTH_PNT_MGHousing2TMAir_Heat_Resi_KpW
  Divide : Product  Inputs=*/
  Gain : Gain  Gain=-1
  Gain1 : Gain
  PHI_MG2Air_Resi1_W : Outport
  PHI_MGHousing_Resi5_W : Outport  Port=2
  wires:
  Constant/1 -> Divide/2
  Add/1 -> Divide/1
  Divide/1 -> Gain1/1, Gain/1
  Gain/1 -> PHI_MGHousing_Resi5_W/1
  T_MGHousing_Resi5_K/1 -> Add/1
  T_MG2Air_Resi1_K/1 -> Add/2
  Gain1/1 -> PHI_MG2Air_Resi1_W/1

== system EV_thermal_charger_2015a_jmaab_Can01/Vehicle/ELTH/ELTH_PNT/MGTH_PNT/MGHousing_Heat_Capacity ==
  PHI_MGHousing2_W : Inport
  PHI_MGHousing3_W : Inport  Port=2
  PHI_MGHousing4_W : Inport  Port=3
  Temp_ini : Inport  Port=4
  PHI_MGHousing1_W : Inport  Port=5
  PHI_MGHousing5_W : Inport  Port=6
  Add : Sum  Inputs=+++++
  Add1 : Sum
  Constant : Constant  Value=ELTH_PNT_MGHousing_Heat_Capa_JpK
  Divide : Product  Inputs=/*
  Integrator : Integrator
  degC->K : Subsystem
  T_MGHousing2_K : Outport
  T_MGHousing3_K : Outport  Port=2
  T_MGHousing4_K : Outport  Port=3
  T_MGHousing5_K : Outport  Port=4
  T_MGHousing1_K : Outport  Port=5
  wires:
  PHI_MGHousing1_W/1 -> Add/1
  Constant/1 -> Divide/1
  Add/1 -> Divide/2
  Divide/1 -> Integrator/1
  Temp_ini/1 -> degC->K/1(degC)
  Integrator/1 -> Add1/2
  Add1/1 -> T_MGHousing1_K/1, T_MGHousing2_K/1, T_MGHousing5_K/1, T_MGHousing3_K/1, T_MGHousing4_K/1
  degC->K/1(K) -> Add1/1
  PHI_MGHousing2_W/1 -> Add/2
  PHI_MGHousing3_W/1 -> Add/5
  PHI_MGHousing4_W/1 -> Add/4
  PHI_MGHousing5_W/1 -> Add/3

== system EV_thermal_charger_2015a_jmaab_Can01/Vehicle/ELTH/ELTH_PNT/MGTH_PNT/PTTH2MGHousing_Heat_Resistance ==
  T_MGHousing_Resi2_K : Inport
  T_PTTH_Resi2_K : Inport  Port=2
  Add : Sum  Inputs=+-
  Constant : Constant  Value=ELTH_PNT_PTTH2MGHousing_Heat_Resi_KpW
  Divide : Product  Inputs=*/
  Gain : Gain  Gain=-1
  Gain1 : Gain
  PHI_MGHousing_Resi2_W : Outport
  PHI_PTTH_Resi2_W : Outport  Port=2
  wires:
  Constant/1 -> Divide/2
  Add/1 -> Divide/1
  Divide/1 -> Gain1/1, Gain/1
  Gain/1 -> PHI_PTTH_Resi2_W/1
  T_PTTH_Resi2_K/1 -> Add/1
  T_MGHousing_Resi2_K/1 -> Add/2
  Gain1/1 -> PHI_MGHousing_Resi2_W/1

== system EV_thermal_charger_2015a_jmaab_Can01/Vehicle/ELTH/ELTH_PNT/RD_PNT/INV2Coolant_Heat_Resistance1 ==
  Qv_Coolant_m3ps : Inport
  T_INVTH_Resi_K : Inport  Port=2
  T_Coolant_Resi_K : Inport  Port=3
  1-D Lookup Table : Lookup_n-D  NumberOfTableDimensions=1  BreakpointsForDimension1=ELTH_PNT_INV2Coolant_Heat_Resi_x_qv_Coolant  Table=ELTH_PNT_INV2Coolant_Heat_Resi_KpW  InternalRulePriority=Speed  RndMeth=Simplest  InputSameDT=on
  Add : Sum  Inputs=+-
  Divide : Product  Inputs=*/
  Gain : Gain  Gain=-1
  Gain1 : Gain
  PHI_Coolant_Resi_W : Outport
  PHI_INVTH_Resi_W : Outport  Port=2
  wires:
  1-D Lookup Table/1 -> Divide/2
  Add/1 -> Divide/1
  Divide/1 -> Gain1/1, Gain/1
  T_Coolant_Resi_K/1 -> Add/2
  T_INVTH_Resi_K/1 -> Add/1
  Gain/1 -> PHI_INVTH_Resi_W/1
  Gain1/1 -> PHI_Coolant_Resi_W/1
  Qv_Coolant_m3ps/1 -> 1-D Lookup Table/1

== system EV_thermal_charger_2015a_jmaab_Can01/Vehicle/ELTH/ELTH_PNT/RD_PNT/K->degC1 ==
  K : Inport
  Constant2 : Constant  Value=K2degC
  Sum : Sum  Inputs=++|
  degC : Outport
  wires:
  K/1 -> Sum/2
  Constant2/1 -> Sum/1
  Sum/1 -> degC/1

== system EV_thermal_charger_2015a_jmaab_Can01/Vehicle/ELTH/ELTH_PNT/RD_PNT/MG2Coolant_Heat_Resistance ==
  T_Coolant_Resi2_K : Inport
  Qv_Coolant_m3ps : Inport  Port=2
  T_MGTH_Resi2_K : Inport  Port=3
  1-D Lookup Table : Lookup_n-D  NumberOfTableDimensions=1  BreakpointsForDimension1=ELTH_PNT_MG2Coolant_Heat_Resi_x_qv_Coolant  Table=ELTH_PNT_MG2Coolant_Heat_Resi_KpW  InternalRulePriority=Speed  RndMeth=Simplest  InputSameDT=on
  Add : Sum  Inputs=+-
  Divide : Product  Inputs=*/
  Gain : Gain  Gain=-1
  Gain1 : Gain  Gain=+1
  PHI_MGTH_Resi2_W : Outport
  PHI_Coolant_Resi2_W : Outport  Port=2
  wires:
  1-D Lookup Table/1 -> Divide/2
  Add/1 -> Divide/1
  Divide/1 -> Gain1/1, Gain/1
  T_Coolant_Resi2_K/1 -> Add/2
  T_MGTH_Resi2_K/1 -> Add/1
  Gain/1 -> PHI_MGTH_Resi2_W/1
  Gain1/1 -> PHI_Coolant_Resi2_W/1
  Qv_Coolant_m3ps/1 -> 1-D Lookup Table/1

== system EV_thermal_charger_2015a_jmaab_Can01/Vehicle/ELTH/ELTH_PNT/RD_PNT/RDCoolant2Air_Heat_Resistance ==
  T_RD_Air_Resi1_K : Inport
  "RD_PNT_RDCore_Heat_Resi_KpW " : Inport  Port=2
  T_RDCoolant_Resi2_K : Inport  Port=3
  Add : Sum  Inputs=+-
  Divide : Product  Inputs=*/
  Gain : Gain  Gain=-1
  Gain1 : Gain
  PHI_RD_Air_Resi1_W : Outport
  PHI_RDCoolant_Resi2_W : Outport  Port=2
  wires:
  "RD_PNT_RDCore_Heat_Resi_KpW "/1 -> Divide/2
  Add/1 -> Divide/1
  Divide/1 -> Gain1/1, Gain/1
  Gain/1 -> PHI_RDCoolant_Resi2_W/1
  T_RDCoolant_Resi2_K/1 -> Add/1
  T_RD_Air_Resi1_K/1 -> Add/2
  Gain1/1 -> PHI_RD_Air_Resi1_W/1

== system EV_thermal_charger_2015a_jmaab_Can01/Vehicle/ELTH/ELTH_PNT/RD_PNT/RDCoolant_Heat_Capacity ==
  Temp_ini : Inport
  PHI_RDCoolant1_W : Inport  Port=2
  PHI_RDCoolant2_W : Inport  Port=3
  Add : Sum
  Add1 : Sum
  Constant : Constant  Value=ELTH_PNT_RDCoolant_Heat_Capa_JpK
  Divide : Product  Inputs=/*
  Integrator : Integrator
  degC->K : Subsystem
  T_RDCoolant2_K : Outport
  T_RDCoolant1_K : Outport  Port=2
  wires:
  PHI_RDCoolant2_W/1 -> Add/2
  PHI_RDCoolant1_W/1 -> Add/1
  Constant/1 -> Divide/1
  Add/1 -> Divide/2
  Divide/1 -> Integrator/1
  Temp_ini/1 -> degC->K/1(degC)
  Integrator/1 -> Add1/2
  Add1/1 -> T_RDCoolant2_K/1, T_RDCoolant1_K/1
  degC->K/1(K) -> Add1/1

== system EV_thermal_charger_2015a_jmaab_Can01/Vehicle/ELTH/ELTH_PNT/RD_PNT/RD_Core_Heat_Resi_Calc ==
  note: ラジエターファンの動作で
      | 発生する風速
  note: 車両の走行によって
      | ラジエターグリルに発生する風速
  note: ラジエターファンの動作で
      | ラジエターコアに当たる風量
  note: 車両の走行によって
      | ラジエターコアに当たる風量
  ELTH_PNT_Voltage_RDFan_V : Inport
  v_VL_PNT_mps : Inport  Port=2
  1-D Lookup Table : Lookup_n-D  NumberOfTableDimensions=1  BreakpointsForDimension1=ELTH_PNT_RDCore_Heat_Resi_KpW_x_Wind_m3ps  Table=ELTH_PNT_RDCore_Heat_Resi_KpW  InternalRulePriority=Speed  RndMeth=Simplest  InputSameDT=on
  1-D Lookup Table1 : Lookup_n-D  NumberOfTableDimensions=1  BreakpointsForDimension1=ELTH_PNT_v_RDFan_Wind_vel_mps_x_V_RDFan  Table=ELTH_PNT_v_RDFan_Wind_vel_mps  InternalRulePriority=Speed  RndMeth=Simplest  InputSameDT=on
  1-D Lookup Table2 : Lookup_n-D  NumberOfTableDimensions=1  BreakpointsForDimension1=ELTH_PNT_RDCore_Heat_Resi_KpW_x_Wind_m3ps  Table=ELTH_PNT_RDCore_Heat_Resi_KpW  InternalRulePriority=Speed  RndMeth=Simplest  InputSameDT=on
  Abs : Abs
  Add : Sum
  Constant : Constant  Value=ELTH_PNT_RDFan_area_m2
  Constant1 : Constant  Value=ELTH_PNT_RDGrill_area_m2
  Product : Product
  Product1 : Product
  gain1 : Gain  Commented=through  Gain=kmph2mps
  "ELTH_PNT_RDCore_Heat_Resi_KpW " : Outport
  ELTH_PNT_AirconCore_Heat_Resi_KpW : Outport  Port=2
  wires:
  ELTH_PNT_Voltage_RDFan_V/1 -> 1-D Lookup Table1/1
  Constant/1 -> Product/2
  v_VL_PNT_mps/1 -> gain1/1
  Constant1/1 -> Product1/2
  Product/1 -> Add/1
  Product1/1 -> Add/2
  Add/1 -> Abs/1
  1-D Lookup Table/1 -> "ELTH_PNT_RDCore_Heat_Resi_KpW "/1
  Abs/1 -> 1-D Lookup Table2/1, 1-D Lookup Table/1
  1-D Lookup Table1/1 -> Product/1
  gain1/1 -> Product1/1
  1-D Lookup Table2/1 -> ELTH_PNT_AirconCore_Heat_Resi_KpW/1

== system EV_thermal_charger_2015a_jmaab_Can01/Vehicle/ELTH/ELTH_PNT/RD_PNT/Water_Pump ==
  ELTH_PNT_Voltage_WP_V : Inport
  1-D Lookup Table : Lookup_n-D  NumberOfTableDimensions=1  BreakpointsForDimension1=ELTH_PNT_Qv_Water_Pump_x_V_WP  Table=ELTH_PNT_Qv_Water_Pump_m3ps  InternalRulePriority=Speed  RndMeth=Simplest  InputSameDT=on
  Qv_Coolant_m3ps : Outport
  wires:
  ELTH_PNT_Voltage_WP_V/1 -> 1-D Lookup Table/1
  1-D Lookup Table/1 -> Qv_Coolant_m3ps/1

== system EV_thermal_charger_2015a_jmaab_Can01/Vehicle/BTTH/BTTH_PNT/BB_PNT/BTBlock_Heat_Capacity/degC->K ==
  degC : Inport
  Constant2 : Constant  Value=degC2K
  Sum : Sum  Inputs=++|
  K : Outport
  wires:
  degC/1 -> Sum/2
  Constant2/1 -> Sum/1
  Sum/1 -> K/1

== system EV_thermal_charger_2015a_jmaab_Can01/Vehicle/BTTH/BTTH_PNT/BC_PNT/BTCells_Heat_Capacity/degC->K ==
  degC : Inport
  Constant2 : Constant  Value=degC2K
  Sum : Sum  Inputs=++|
  K : Outport
  wires:
  degC/1 -> Sum/2
  Constant2/1 -> Sum/1
  Sum/1 -> K/1

== system EV_thermal_charger_2015a_jmaab_Can01/Vehicle/BTTH/BTTH_PNT/BH_PNT/BT_Heater_Heat_Capacity/degC->K ==
  degC : Inport
  Constant2 : Constant  Value=degC2K
  Sum : Sum  Inputs=++|
  K : Outport
  wires:
  degC/1 -> Sum/2
  Constant2/1 -> Sum/1
  Sum/1 -> K/1

== system EV_thermal_charger_2015a_jmaab_Can01/Vehicle/CATH/CATH_PNT/CABIN/CABIN_AIR/degC->K ==
  degC : Inport
  Constant2 : Constant  Value=degC2K
  Sum : Sum  Inputs=++|
  K : Outport
  wires:
  degC/1 -> Sum/2
  Constant2/1 -> Sum/1
  Sum/1 -> K/1

== system EV_thermal_charger_2015a_jmaab_Can01/Vehicle/CATH/CATH_PNT/CABIN/GLASS/CABIN_Glass_Heat_Capacity ==
  Temp_ini : Inport
  PHI_CABIN_Glass1_W : Inport  Port=2
  PHI_CABIN_Glass2_W : Inport  Port=3
  Add : Sum
  Add1 : Sum
  Constant : Constant  Value=CATH_PNT_Glass_Heat_Capa_JpK
  Divide : Product  Inputs=/*
  Integrator : Integrator  LowerSaturationLimit=0
  degC->K : Subsystem
  T_CABIN_Glass2_K : Outport
  T_CABIN_Glass1_K : Outport  Port=2
  wires:
  PHI_CABIN_Glass2_W/1 -> Add/2
  PHI_CABIN_Glass1_W/1 -> Add/1
  Constant/1 -> Divide/1
  Add/1 -> Divide/2
  Divide/1 -> Integrator/1
  Temp_ini/1 -> degC->K/1(degC)
  Integrator/1 -> Add1/2
  Add1/1 -> T_CABIN_Glass1_K/1, T_CABIN_Glass2_K/1
  degC->K/1(K) -> Add1/1

== system EV_thermal_charger_2015a_jmaab_Can01/Vehicle/CATH/CATH_PNT/CABIN/GLASS/CABIN_Glass_Heat_Resistance ==
  note: ガラスの熱抵抗
      | の半分
  V_wind : Inport
  T_CABIN_Glass_Resi1_K : Inport  Port=2
  T_CABIN_Glass_Resi2_K : Inport  Port=3
  Add : Sum  Inputs=+-
  Constant1 : Constant  Value=CATH_PNT_CABIN_Glass_S_m2
  Constant2 : Constant  Value=CATH_PNT_Glass_emissivity
  Divide : Product  Inputs=/*
  Gain : Gain  Gain=-1
  Gain1 : Gain
  Heat_Resistance_Calc : Subsystem
  R3m2 : Constant  Value=CATH_PNT_Glass_Heat_Resi_m2KpW /2
  PHI_CABIN_Glass_Resi1_W : Outport
  PHI_CABIN_Glass_Resi2_W : Outport  Port=2
  wires:
  Add/1 -> Divide/2
  Divide/1 -> Gain/1, Gain1/1
  Gain/1 -> PHI_CABIN_Glass_Resi2_W/1
  Gain1/1 -> PHI_CABIN_Glass_Resi1_W/1
  T_CABIN_Glass_Resi2_K/1 -> Add/1, Heat_Resistance_Calc/6(T_Glass_center_K)
  T_CABIN_Glass_Resi1_K/1 -> Heat_Resistance_Calc/5(T_In1_K), Add/2
  Heat_Resistance_Calc/1(R_total) -> Divide/1
  V_wind/1 -> Heat_Resistance_Calc/1(V_wind_mps)
  Constant1/1 -> Heat_Resistance_Calc/2(S_Heat_Conduction_m2)
  Constant2/1 -> Heat_Resistance_Calc/3(emissivity)
  R3m2/1 -> Heat_Resistance_Calc/4(wall_heat_resi)

== system EV_thermal_charger_2015a_jmaab_Can01/Vehicle/CATH/CATH_PNT/CABIN/GLASS/CABIN_Glass_Heat_Resistance1 ==
  note: ガラスの熱抵抗
      | の半分
  V_wind : Inport
  T_CABIN_Glass_Resi4_K : Inport  Port=2
  T_CABIN_Glass_Resi3_K : Inport  Port=3
  Add : Sum  Inputs=+-
  Constant1 : Constant  Value=CATH_PNT_CABIN_Glass_S_m2
  Constant2 : Constant  Value=CATH_PNT_Glass_emissivity
  Divide : Product  Inputs=/*
  Gain : Gain  Gain=-1
  Gain1 : Gain
  Heat_Resistance_Calc : Subsystem
  R3m2 : Constant  Value=CATH_PNT_Glass_Heat_Resi_m2KpW /2
  PHI_CABIN_Glass_Resi4_W : Outport
  PHI_CABIN_Glass_Resi3_W : Outport  Port=2
  wires:
  Heat_Resistance_Calc/1(R_total) -> Divide/1
  Add/1 -> Divide/2
  Divide/1 -> Gain1/1, Gain/1
  Gain/1 -> PHI_CABIN_Glass_Resi4_W/1
  T_CABIN_Glass_Resi4_K/1 -> Add/1, Heat_Resistance_Calc/5(T_In1_K)
  T_CABIN_Glass_Resi3_K/1 -> Heat_Resistance_Calc/6(T_Glass_center_K), Add/2
  Gain1/1 -> PHI_CABIN_Glass_Resi3_W/1
  V_wind/1 -> Heat_Resistance_Calc/1(V_wind_mps)
  Constant1/1 -> Heat_Resistance_Calc/2(S_Heat_Conduction_m2)
  Constant2/1 -> Heat_Resistance_Calc/3(emissivity)
  R3m2/1 -> Heat_Resistance_Calc/4(wall_heat_resi)

== system EV_thermal_charger_2015a_jmaab_Can01/Vehicle/CATH/CATH_PNT/CABIN/WALL/CABIN_Wall_Heat_Capacity ==
  Temp_ini : Inport
  PHI_CABIN_Wall1_W : Inport  Port=2
  PHI_CABIN_Wall2_W : Inport  Port=3
  Add : Sum
  Add1 : Sum
  Constant : Constant  Value=CATH_PNT_Wall_Heat_Capa_JpK
  Divide : Product  Inputs=/*
  Integrator : Integrator
  degC->K : Subsystem
  T_CABIN_Wall2_K : Outport
  T_CABIN_Wall1_K : Outport  Port=2
  wires:
  PHI_CABIN_Wall2_W/1 -> Add/2
  PHI_CABIN_Wall1_W/1 -> Add/1
  Constant/1 -> Divide/1
  Add/1 -> Divide/2
  Divide/1 -> Integrator/1
  Temp_ini/1 -> degC->K/1(degC)
  Integrator/1 -> Add1/2
  Add1/1 -> T_CABIN_Wall2_K/1, T_CABIN_Wall1_K/1
  degC->K/1(K) -> Add1/1

== system EV_thermal_charger_2015a_jmaab_Can01/Vehicle/CATH/CATH_PNT/CABIN/WALL/CABIN_Wall_Heat_Resistance ==
  note: 不透明壁の熱抵抗
      | の半分
  V_wind : Inport
  T_Wall_Resi1_K : Inport  Port=2
  T_Wall_Resi2_K : Inport  Port=3
  Add : Sum  Inputs=+-
  Constant1 : Constant  Value=CATH_PNT_CABIN_Wall_S_m2
  Constant2 : Constant  Value=CATH_PNT_Wall_emissivity
  Divide : Product  Inputs=/*
  Gain : Gain  Gain=-1
  Gain1 : Gain
  Heat_Resistance_Calc : Subsystem
  R3m2 : Constant  Value=CATH_PNT_Wall_Heat_Resi_m2KpW /2
  PHI_Wall_Resi1_W : Outport
  PHI_Wall_Resi2_W : Outport  Port=2
  wires:
  Add/1 -> Divide/2
  Divide/1 -> Gain1/1, Gain/1
  Gain/1 -> PHI_Wall_Resi2_W/1
  Gain1/1 -> PHI_Wall_Resi1_W/1
  T_Wall_Resi1_K/1 -> Add/2, Heat_Resistance_Calc/5(T_In1_K)
  Heat_Resistance_Calc/1(R_total) -> Divide/1
  V_wind/1 -> Heat_Resistance_Calc/1(V_wind_mps)
  Constant1/1 -> Heat_Resistance_Calc/2(S_Heat_Conduction_m2)
  Constant2/1 -> Heat_Resistance_Calc/3(emissivity)
  R3m2/1 -> Heat_Resistance_Calc/4(wall_heat_resi)
  T_Wall_Resi2_K/1 -> Heat_Resistance_Calc/6(T_Glass_center_K), Add/1

== system EV_thermal_charger_2015a_jmaab_Can01/Vehicle/CATH/CATH_PNT/CABIN/WALL/CABIN_Wall_Heat_Resistance1 ==
  note: 不透明壁の熱抵抗
      | の半分
  V_wind : Inport
  T_CABIN_Wall_Resi2_K : Inport  Port=2
  T_CABIN_Wall_Resi1_K : Inport  Port=3
  Add : Sum  Inputs=+-
  Constant1 : Constant  Value=CATH_PNT_CABIN_Wall_S_m2
  Constant2 : Constant  Value=CATH_PNT_Wall_emissivity
  Divide : Product  Inputs=/*
  Gain : Gain  Gain=-1
  Gain1 : Gain
  Heat_Resistance_Calc : Subsystem
  R3m2 : Constant  Value=CATH_PNT_Wall_Heat_Resi_m2KpW /2
  PHI_CABIN_Wall_Resi2_W : Outport
  PHI_CABIN_Wall_Resi1_W : Outport  Port=2
  wires:
  Add/1 -> Divide/2
  Divide/1 -> Gain1/1, Gain/1
  Gain1/1 -> PHI_CABIN_Wall_Resi1_W/1
  T_CABIN_Wall_Resi2_K/1 -> Add/1, Heat_Resistance_Calc/5(T_In1_K)
  T_CABIN_Wall_Resi1_K/1 -> Add/2, Heat_Resistance_Calc/6(T_Glass_center_K)
  Heat_Resistance_Calc/1(R_total) -> Divide/1
  V_wind/1 -> Heat_Resistance_Calc/1(V_wind_mps)
  Constant1/1 -> Heat_Resistance_Calc/2(S_Heat_Conduction_m2)
  Constant2/1 -> Heat_Resistance_Calc/3(emissivity)
  R3m2/1 -> Heat_Resistance_Calc/4(wall_heat_resi)
  Gain/1 -> PHI_CABIN_Wall_Resi2_W/1

== system EV_thermal_charger_2015a_jmaab_Can01/Vehicle/CATH/CATH_PNT/HVAC/Aircon/Aircon_Indoor_Unit_Heat_Capacity1 ==
  Temp_ini : Inport
  PHI_Aircon_Indoor3_W : Inport  Port=2
  PHI_Aircon_Indoor2_W : Inport  Port=3
  Add : Sum
  Add1 : Sum
  Constant : Constant  Value=CATH_PNT_Aircon_Indoor_Unit_Heat_Capa_JpK
  Divide : Product  Inputs=/*
  Integrator : Integrator
  degC->K : Subsystem
  T_Aircon_Indoor2_K : Outport
  T_Aircon_Indoor3_K : Outport  Port=2
  wires:
  PHI_Aircon_Indoor2_W/1 -> Add/2
  PHI_Aircon_Indoor3_W/1 -> Add/1
  Constant/1 -> Divide/1
  Add/1 -> Divide/2
  Divide/1 -> Integrator/1
  Temp_ini/1 -> degC->K/1(degC)
  Integrator/1 -> Add1/2
  Add1/1 -> T_Aircon_Indoor2_K/1, T_Aircon_Indoor3_K/1
  degC->K/1(K) -> Add1/1

== system EV_thermal_charger_2015a_jmaab_Can01/Vehicle/CATH/CATH_PNT/HVAC/Aircon/Aircon_Outdoor_Unit_Heat_Capacity ==
  Temp_ini : Inport
  PHI_Aircon_Outdoor3_W : Inport  Port=2
  PHI_Aircon_Outdoor2_W : Inport  Port=3
  Add : Sum
  Add1 : Sum
  Constant : Constant  Value=CATH_PNT_Aircon_Outdoor_Unit_Heat_Capa_JpK
  Divide : Product  Inputs=/*
  Integrator : Integrator
  degC->K : Subsystem
  T_Aircon_Outdoor2_K : Outport
  T_Aircon_Outdoor3_K : Outport  Port=2
  wires:
  PHI_Aircon_Outdoor2_W/1 -> Add/2
  PHI_Aircon_Outdoor3_W/1 -> Add/1
  Constant/1 -> Divide/1
  Add/1 -> Divide/2
  Divide/1 -> Integrator/1
  Temp_ini/1 -> degC->K/1(degC)
  Integrator/1 -> Add1/2
  Add1/1 -> T_Aircon_Outdoor3_K/1, T_Aircon_Outdoor2_K/1
  degC->K/1(K) -> Add1/1

== system EV_thermal_charger_2015a_jmaab_Can01/Vehicle/CATH/CATH_PNT/HVAC/Aircon/K->degC ==
  K : Inport
  Constant2 : Constant  Value=K2degC
  Sum : Sum  Inputs=++|
  degC : Outport
  wires:
  K/1 -> Sum/2
  Constant2/1 -> Sum/1
  Sum/1 -> degC/1

== system EV_thermal_charger_2015a_jmaab_Can01/Vehicle/CATH/CATH_PNT/HVAC/Aircon/K->degC1 ==
  K : Inport
  Constant2 : Constant  Value=K2degC
  Sum : Sum  Inputs=++|
  degC : Outport
  wires:
  K/1 -> Sum/2
  Constant2/1 -> Sum/1
  Sum/1 -> degC/1

== system EV_thermal_charger_2015a_jmaab_Can01/Vehicle/CATH/CATH_PNT/HVAC/Aircon/Switching_Air_Conditioning_Circuit ==
  note: コンデンサ側熱流量
  note: ヒートポンプパワー＞0 → 車室への熱量＞0 ＝暖房
      |
      | ヒートポンプ パワー＜0 → 車室への熱量＜0 ＝冷房
  note: エバポレータ側熱流量
  note: コンプレッサ消費電力
  note: 冷暖房判定で
      | エバポレータ・コンデンサ切替
  V_Compressor_V : Inport
  P_Heatpomp_Power : Inport  Port=2
  T_Aircon_Indoor4_K : Inport  Port=3
  T_Aircon_Outdoor4_K : Inport  Port=4
  Abs : Abs
  Add1 : Sum
  Compare To Zero : simulink/Logic and Bit Operations/Compare To Zero  relop=<  OutDataTypeStr=boolean
  Constant1 : Constant  Value=CATH_PNT_COP_Aircon
  Divide_0wari1 : METI_Lib_vehicle_model/Divide_0wari
  Gain : Gain  Gain=-1
  Gain1 : Gain  Gain=-1
  Product2 : Product
  Switch : Switch  Criteria=u2 > Threshold
  Switch1 : Switch  Criteria=u2 > Threshold
  Terminator : Terminator
  Terminator1 : Terminator
  I_Compressor_A : Outport
  PHI_Aircon_Outdoor4_W : Outport  Port=2
  PHI_Aircon_Indoor4_W : Outport  Port=3
  wires:
  Compare To Zero/1 -> Switch/2, Switch1/2
  P_Heatpomp_Power/1 -> Abs/1, Compare To Zero/1
  Add1/1 -> Switch1/1, Switch/3
  Switch/1 -> PHI_Aircon_Indoor4_W/1
  Switch1/1 -> PHI_Aircon_Outdoor4_W/1
  Gain/1 -> Switch1/3, Switch/1
  Product2/1 -> Add1/1, Gain/1
  Constant1/1 -> Product2/2
  Abs/1 -> Product2/1, Divide_0wari1/1, Add1/2
  T_Aircon_Indoor4_K/1 -> Terminator/1
  T_Aircon_Outdoor4_K/1 -> Terminator1/1
  V_Compressor_V/1 -> Divide_0wari1/2
  Divide_0wari1/1 -> Gain1/1
  Gain1/1 -> I_Compressor_A/1

== system EV_thermal_charger_2015a_jmaab_Can01/Vehicle/CATH/CATH_PNT/HVAC/PTC_Heater1/K->degC ==
  K : Inport
  Constant2 : Constant  Value=K2degC
  Sum : Sum  Inputs=++|
  degC : Outport
  wires:
  K/1 -> Sum/2
  Constant2/1 -> Sum/1
  Sum/1 -> degC/1

== system EV_thermal_charger_2015a_jmaab_Can01/Vehicle/CATH/CATH_PNT/HVAC/PTC_Heater1/PTC_Heater ==
  P_PTC_Heater_Power : Inport
  V_PTC_Heater4_V : Inport  Port=2
  T_PTC_Heater4_K : Inport  Port=3
  Divide_0wari : METI_Lib_vehicle_model/Divide_0wari
  Gain : Gain  Gain=-1
  Terminator : Terminator
  PHI_PTC_Heater4_W : Outport
  I_PTC_Heater4_A : Outport  Port=2
  wires:
  Divide_0wari/1 -> Gain/1
  P_PTC_Heater_Power/1 -> PHI_PTC_Heater4_W/1, Divide_0wari/1
  V_PTC_Heater4_V/1 -> Divide_0wari/2
  Gain/1 -> I_PTC_Heater4_A/1
  T_PTC_Heater4_K/1 -> Terminator/1

== system EV_thermal_charger_2015a_jmaab_Can01/Vehicle/CATH/CATH_PNT/HVAC/PTC_Heater1/PTC_Heater_Heat_Capacity ==
  Temp_ini : Inport
  PHI_PTC_Heater3_W : Inport  Port=2
  PHI_PTC_Heater2_W : Inport  Port=3
  Add : Sum
  Add1 : Sum
  Constant : Constant  Value=CATH_PNT_PTC_Heater_Heat_Capa_JpK
  Divide : Product  Inputs=/*
  Integrator : Integrator
  degC->K : Subsystem
  T_PTC_Heater2_K : Outport
  T_PTC_Heater3_K : Outport  Port=2
  wires:
  PHI_PTC_Heater2_W/1 -> Add/2
  PHI_PTC_Heater3_W/1 -> Add/1
  Constant/1 -> Divide/1
  Add/1 -> Divide/2
  Divide/1 -> Integrator/1
  Temp_ini/1 -> degC->K/1(degC)
  Integrator/1 -> Add1/2
  Add1/1 -> T_PTC_Heater3_K/1, T_PTC_Heater2_K/1
  degC->K/1(K) -> Add1/1

== system EV_thermal_charger_2015a_jmaab_Can01/Vehicle/CATH/CATH_PNT/Seat_Heater/SeatHT_Heat_Capacity/degC->K ==
  degC : Inport
  Constant2 : Constant  Value=degC2K
  Sum : Sum  Inputs=++|
  K : Outport
  wires:
  degC/1 -> Sum/2
  Constant2/1 -> Sum/1
  Sum/1 -> K/1

== system EV_thermal_charger_2015a_jmaab_Can01/Vehicle/CNT/CATH_CNT/CATH_CNT/Calc_Temp_Blowout/FB ==
  T_diff_temp_degC : Inport
  Constant : Constant  Value=CATH_CNT_PGain_Temp_blowout
  Product : Product
  Q_FB : Outport
  wires:
  T_diff_temp_degC/1 -> Product/1
  Product/1 -> Q_FB/1
  Constant/1 -> Product/2

== system EV_thermal_charger_2015a_jmaab_Can01/Vehicle/CNT/CATH_CNT/CATH_CNT/Calc_Temp_Blowout/FF1 ==
  note: [m2K/W]
  note: ユルゲスの実験式による
      | 対流の熱伝達率[W/m2K]を逆数にして
      | 熱抵抗[m2K/W]にしたもの
  note: [m2K/W]
  note: ユルゲスの実験式による
      | 対流の熱伝達率[W/m2K]を逆数にして
      | 熱抵抗[m2K/W]にしたもの
  note: 室内の風速
  T_Outside_temp_degC : Inport
  T_CABIN_AIR_temp_degC : Inport  Port=2
  v_VL_PNT_kmph : Inport  Port=3
  Abs : Abs
  Add : Sum
  Air_Convection_Heat_Resi : Lookup_n-D  NumberOfTableDimensions=1  BreakpointsForDimension1=CATH_PNT_Air_Convection_Heat_Resi_x_mps  Table=CATH_PNT_Air_Convection_Heat_Resi_KpW  InternalRulePriority=Speed  RndMeth=Simplest  InputSameDT=on
  Air_Convection_Heat_Resi1 : Lookup_n-D  NumberOfTableDimensions=1  BreakpointsForDimension1=CATH_PNT_Air_Convection_Heat_Resi_x_mps  Table=CATH_PNT_Air_Convection_Heat_Resi_KpW  InternalRulePriority=Speed  RndMeth=Simplest  InputSameDT=on
  Constant1 : Constant  Value=CATH_PNT_CABIN_Glass_S_m2
  Constant2 : Constant  Value=CATH_PNT_CABIN_Glass_S_m2
  Constant3 : Constant
  Divide : Product  Inputs=*/
  Divide1 : Product  Inputs=*/
  Divide2 : Product  Inputs=*/
  Subtract : Sum  Inputs=-+
  kmph2mps : Gain  Gain=kmph2mps
  Q_Heat_Transfar : Outport
  wires:
  T_Outside_temp_degC/1 -> Subtract/1
  T_CABIN_AIR_temp_degC/1 -> Subtract/2
  Divide1/1 -> Q_Heat_Transfar/1
  Air_Convection_Heat_Resi/1 -> Divide/1
  Abs/1 -> Air_Convection_Heat_Resi/1
  Constant1/1 -> Divide/2
  v_VL_PNT_kmph/1 -> kmph2mps/1
  Subtract/1 -> Divide1/1
  Air_Convection_Heat_Resi1/1 -> Divide2/1
  Constant3/1 -> Air_Convection_Heat_Resi1/1
  Constant2/1 -> Divide2/2
  Divide/1 -> Add/1
  Divide2/1 -> Add/2
  Add/1 -> Divide1/2
  kmph2mps/1 -> Abs/1

== system EV_thermal_charger_2015a_jmaab_Can01/Vehicle/CNT/CHG_CNT/CHG_CNT/Charge_Current_calc/Initial_Charge ==
  In1 : Inport
  Action Port : ActionPort  ActionType=elseif
  Out1 : Outport
  wires:
  In1/1 -> Out1/1

== system EV_thermal_charger_2015a_jmaab_Can01/Vehicle/CNT/CHG_CNT/CHG_CNT/Charge_Current_calc/Negotiation_time ==
  Action Port : ActionPort  ActionType=then
  Constant : Constant  Value=0
  Out1 : Outport
  wires:
  Constant/1 -> Out1/1

== system EV_thermal_charger_2015a_jmaab_Can01/Vehicle/CNT/CHG_CNT/CHG_CNT/Charge_Current_calc/Normal_Charge ==
  note: 一定電流充電モード（CC)
      | 一定電力充電モード（CP)
      | 一定電圧充電モード（CV)
      | の三者で目標電流値を算出し、
      | その中で最も小さい電流値だったものを採用する。
  Maximum_Charge_Current_A : Inport
  Maximum_Charge_Power_W : Inport  Port=2
  Maximum_Charge_Voltage_V : Inport  Port=3
  Battery_Voltage_V : Inport  Port=4
  SOC_HiBatt : Inport  Port=5
  Maximum_Hi_Batt_SOC : Inport  Port=6
  Action Port : ActionPort  ActionType=else
  Constant_Current_Charge : Subsystem
  Constant_Power_Charge : Subsystem
  Constant_Voltage_Charge : Subsystem
  Memory : Memory
  MinMax : MinMax  Inputs=3
  Relational Operator : RelationalOperator  Operator===  OutDataTypeStr=boolean
  Current_tgt : Outport
  wires:
  Maximum_Charge_Current_A/1 -> Constant_Current_Charge/1(Maximum_Charge_Current_A), Constant_Voltage_Charge/1(Maximum_Charge_Current_A)
  MinMax/1 -> Relational Operator/1, Current_tgt/1
  Maximum_Charge_Power_W/1 -> Constant_Power_Charge/1(Maximum_Charge_Power_W)
  Constant_Current_Charge/1(Current_tgt) -> MinMax/1
  Battery_Voltage_V/1 -> Constant_Power_Charge/2(Battery_Voltage_V), Constant_Voltage_Charge/4(Battery_Voltage_V)
  Constant_Power_Charge/1(Current_tgt) -> MinMax/2
  Constant_Voltage_Charge/1(Current_tgt) -> Relational Operator/2, MinMax/3
  Memory/1 -> Constant_Voltage_Charge/5(old_mode)
  Relational Operator/1 -> Memory/1
  Maximum_Hi_Batt_SOC/1 -> Constant_Voltage_Charge/3(Maximum_Hi_Batt_SOC)
  Maximum_Charge_Voltage_V/1 -> Constant_Voltage_Charge/2(Maximum_Charge_Voltage_V)
  SOC_HiBatt/1 -> Constant_Current_Charge/2(SOC_HiBatt)

== system EV_thermal_charger_2015a_jmaab_Can01/Vehicle/CNT/VCU_CNT/VCU_CNT/ReGenerativeBrake_Calc/ReBrake_Limit_Lowspeed ==
  note: 車速＞回生ブレーキ打ち切り開始速度 の時 出力＝1（回生トルク100%有効）
      |
      | 車速＜回生ブレーキ打ち切り終了速度 の時 出力＝0（回生トルク無効）
      |
      | 開始速度＞車速＞終了速度 の時 出力＝0～1（回生トルクの有効度合いを直線逓減）
  v_VL_PNT_kmph : Inport
  Abs : Abs
  Constant1 : Constant  Value=BK_PNT_Pow_UL
  Constant3 : Constant  Value=BK_PNT_ReGene_vel_limit_UP_kmph
  Constant6 : Constant  Value=BK_PNT_ReGene_vel_limit_DN_kmph
  Constant7 : Constant  Value=0
  Constant8 : Constant
  Divide1 : Product  Inputs=/*
  Gain1 : Gain  Gain=-1
  Product : Product
  Subtract : Sum  Inputs=+-
  Subtract1 : Sum  Inputs=+-
  Subtract2 : Sum  Inputs=+-
  Switch : Switch  Criteria=u2 > Threshold
  Switch1 : Switch  Criteria=u2 > Threshold
  mps2kmph : Gain  Commented=through  Gain=mps2kmph
  F_Brake_limit_lowspeed : Outport
  wires:
  Constant7/1 -> Switch1/3
  Product/1 -> F_Brake_limit_lowspeed/1
  Divide1/1 -> Switch1/1
  Constant3/1 -> Subtract/2, Subtract2/1
  Constant1/1 -> Gain1/1
  Subtract1/1 -> Divide1/2, Switch1/2
  Constant6/1 -> Subtract2/2, Subtract1/2
  Gain1/1 -> Product/1
  Switch1/1 -> Switch/3
  v_VL_PNT_kmph/1 -> mps2kmph/1
  mps2kmph/1 -> Abs/1
  Constant8/1 -> Switch/1
  Subtract/1 -> Switch/2
  Subtract2/1 -> Divide1/1
  Abs/1 -> Subtract1/1, Subtract/1
  Switch/1 -> Product/2
